simulink model "SingularityIdentification"  (R2022a)
settings: Solver=ode4  StartTime=0.0  StopTime=Inf  FixedStep=1/500  RelTol=1e-3
InitFcn:
  | L1 = 0.1400;
  | L2 = 0.3500;
  | L3 = 0.0500;
  | L4 = 0.2500;
  | L5 = 0.1500;
  | l1 = L1;
  | l2 = sqrt(L2^2 + L3^2);
  | l3 = L4 + L5;
  | beta = atan(L3/L2);
  | 
  | home = [0.45; 0; 0.49];
  | default = home;
  | default_w = [0.25; 0.25; 0.1];
  | default_a = [0; 0.375; 0.1];
  | A = [ 0.25; 0.25; 0.01];
  | B = [ 0.25; 0.50; 0.01];
  | C = [-0.25; 0.50; 0.01];
  | D = [-0.25; 0.25; 0.01];
  | 
  | welding_waypoints = [default_w, A, B, C, D, A]' ;
  | assembly_waypoints = [default_a, A, default_a, B, default_a, C, default_a, D]' ;
  | 
  | waypoints = welding_waypoints;
undefined symbols (not defined in the file): HIL, Host
libraries: quarc_library x8
settings Model: ExtModeTrigDuration=10000  Creator=fvranes  LastModifiedBy=lgonzalez
settings SolverCC: AlgebraicLoopSolver=TrustRegion
settings DataIOCC: ReturnWorkspaceOutputs=off
settings DebuggingCC: UnderspecifiedInitializationDetection=Classic  MergeDetectMultiDrivingBlocksExec=none  UnconnectedInputMsg=warning  UnconnectedOutputMsg=warning  UnconnectedLineMsg=warning
settings ModelReferenceCC: PropagateSignalLabelsOutOfModel=off
settings SFSimCC: CustomCodeUndefinedFunction=UseInterfaceOnly

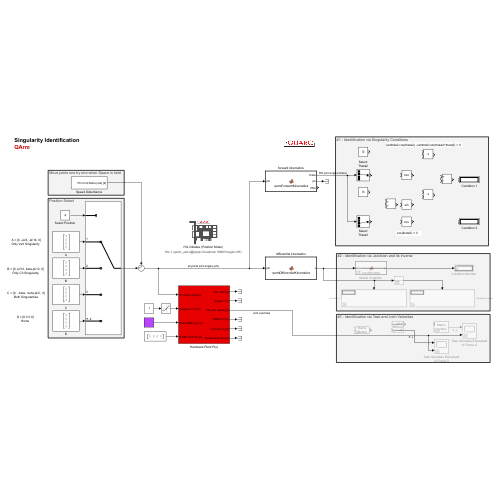
[thumbnail: Simulink's stored preview of the top-level diagram]
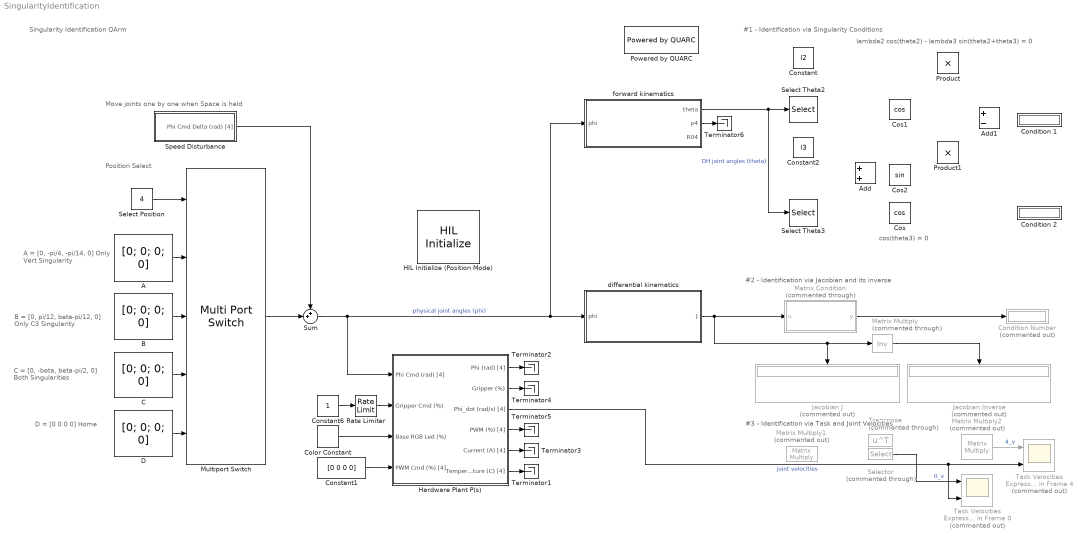
== system SingularityIdentification ==
  note: Move joints one by one when Space is held
  note: Position Select
  note: lambda2 cos(theta2) - lambda3 sin(theta2+theta3) = 0
  note: #1 - Identification via Singularity Conditions
  note: #3 - Identification via Task and Joint Velocities
  note: #2 - Identification via Jacobian and its inverse
  note: A = [0, -pi/4, -pi/14, 0]
      | Only Vert Singularity
  note: B = [0, pi/12, beta-pi/12, 0]
      | Only C3 Singularity
  note: C = [0, -beta, beta-pi/2, 0]
      | Both Singularities
  note: D = [0 0 0 0]
      | Home
  note: cos(theta3) = 0
  note: Singularity Identification
      | QArm
  A : Constant  Value=[0; 0; 0; 0]  VectorParams1D=off
  Add : Sum
  Add1 : Sum  Inputs=+-
  B : Constant  Value=[0; 0; 0; 0]  VectorParams1D=off
  C : Constant  Value=[0; 0; 0; 0]  VectorParams1D=off
  Color Constant : quarc_library/Sources/Signals/Color Constant  color=[0.71765 0.27451 1]
      settings: SourceProductName=QUARC Targets
  Condition 1 : Display
  Condition 2 : Display
  Condition Number : Display  Commented=on
  Constant : Constant  Value=l2
  Constant1 : Constant  Value=[0 0 0 0]
  Constant2 : Constant  Value=l3
  Constant6 : Constant
  Cos : Trigonometry  Operator=cos
  Cos1 : Trigonometry  Operator=cos
  Cos2 : Trigonometry
  D : Constant  Value=[0; 0; 0; 0]  VectorParams1D=off
  HIL Initialize (Position Mode) : quarc_library/Data Acquisition/Generic/Configuration/HIL Initialize  object_name=HIL-1  board_type=qarm_usb  board_number=0@tcpip://localhost:18900?nagle='off'  board_options=j0_mode=0;j1_mode=0;j2_mode=0;j3_mode=0;gripper_mode=0;  exclusive=off  active=on  hardware_clocks=[0]  clock_modes=[]  initial_clock_frequencies=[]  set_clock_params_at_start=off  set_clock_params_at_switch_in=off  set_clock_frequencies_at_start=off  set_clock_frequencies_at_switch_in=off  analog_input_channels=[5:9]  analog_input_configurations=[]  analog_input_maximums=[]  analog_input_minimums=[]  set_analog_input_params_at_start=off  set_analog_input_params_at_switch_in=off  analog_output_channels=[]  analog_output_maximums=inf  analog_output_minimums=-inf  initial_analog_outputs=[0]  final_analog_outputs=[0]  watchdog_analog_outputs=[]  set_analog_output_params_at_start=off  set_analog_output_params_at_switch_in=off  set_analog_outputs_at_start=off  set_analog_outputs_at_switch_in=off  set_analog_outputs_at_terminate=off  set_analog_outputs_at_switch_out=off  set_analog_outputs_on_watchdog=off  digital_input_channels=[]  digital_output_channels=[]  digital_output_configuration=[]  initial_digital_outputs=[0]  final_digital_outputs=[0]  watchdog_digital_outputs=[0]  set_digital_output_params_at_start=off  set_digital_output_params_at_switch_in=off  set_digital_outputs_at_start=off  set_digital_outputs_at_switch_in=off  set_digital_outputs_at_terminate=off  set_digital_outputs_at_switch_out=off  set_digital_outputs_on_watchdog=off  encoder_channels=[]  quadrature=[]  encoder_filter_frequency=[]  initial_encoder_counts=[]  set_encoder_params_at_start=off  set_encoder_params_at_switch_in=off  set_encoder_counts_at_start=off  set_encoder_counts_at_switch_in=off  pwm_channels=[]  pwm_modes=[]  pwm_frequency=[]  pwm_configuration=[]  pwm_alignment=[]  pwm_polarity=[]  pwm_leading_deadband=[]  pwm_trailing_deadband=[]  initial_pwm_outputs=[]  final_pwm_outputs=[]  watchdog_pwm_outputs=[]  set_pwm_params_at_start=off  set_pwm_params_at_switch_in=off  set_pwm_outputs_at_start=off  set_pwm_outputs_at_switch_in=off  set_pwm_outputs_at_terminate=off  set_pwm_outputs_at_switch_out=off  set_pwm_outputs_on_watchdog=off  other_output_channels=[1000:1004 11000:11003 11005:11007]  initial_other_outputs=[zeros(1,9), ones(1,3)]  final_other_outputs=[zeros(1,9), ones(1,3)]  watchdog_other_outputs=zeros(1,12)  set_other_outputs_at_start=off  set_other_outputs_at_switch_in=off  set_other_outputs_at_terminate=on  set_other_outputs_at_switch_out=off  set_other_outputs_on_watchdog=off
  Hardware Plant P(s) : Subsystem
  Jacobian Inverse : Display  Commented=on
  Jacobian J : Display  Commented=on
  Matrix Condition : MATLAB Function  Commented=through  TreatAsAtomicUnit=on
  Matrix Multiply : Product  Commented=through  Inputs=/  Multiplication=Matrix(*)
  Matrix Multiply1 : Product  Commented=on  Multiplication=Matrix(*)
  Matrix Multiply2 : Product  Commented=on  Multiplication=Matrix(*)
  Multiport Switch : MultiPortSwitch  Inputs=4  SaturateOnIntegerOverflow=off  InputSameDT=off
  Powered by QUARC : quarc_library/Logos/Powered by QUARC
  Product : Product
  Product1 : Product
  Rate Limiter : RateLimiter  SampleTimeMode=inherited
  Select Theta2 : Selector  InputPortWidth=4  IndexOptions=Index vector (dialog)  Indices=2  OutputSizes=1
  Select Theta3 : Selector  InputPortWidth=4  IndexOptions=Index vector (dialog)  Indices=3  OutputSizes=1
  Select Position : Constant  Value=4
  Selector : Selector  Commented=through  InputPortWidth=4  IndexOptions=Index vector (dialog)  Indices=[1:3]  OutputSizes=1
  Speed Disturbance : Subsystem
  Sum : Sum  Inputs=++|
  Task Velocities Expressed in Frame 0 : Scope  Commented=on  NumInputPorts=2
  Task Velocities Expressed in Frame 4 : Scope  Commented=on  NumInputPorts=2
  Terminator{1..6} (6 alike) : Terminator
  Transpose : Math  Commented=through  Operator=transpose  SignedPower=on
  differential kinematics : MATLAB Function  TreatAsAtomicUnit=on
  forward kinematics : MATLAB Function  TreatAsAtomicUnit=on
  wires:
  Hardware Plant P(s)/4(PWM (%) [4]) -> Terminator5/1
  Hardware Plant P(s)/3(Phi_dot (rad/s) [4]) -> Task Velocities Expressed in Frame 0/2, Task Velocities Expressed in Frame 4/2  "joint velocities"
  Hardware Plant P(s)/6(Temperature (C) [4]) -> Terminator1/1
  Sum/1 -> Hardware Plant P(s)/1(Phi Cmd (rad) [4]), forward kinematics/1(phi), differential kinematics/1(phi)  "physical joint angles (phi)"
  Rate Limiter/1 -> Hardware Plant P(s)/2(Gripper Cmd (%))
  Hardware Plant P(s)/5(Current (A) [4]) -> Terminator3/1
  Color Constant/1 -> Hardware Plant P(s)/3(Base RGB Led (%))
  Constant1/1 -> Hardware Plant P(s)/4(PWM Cmd (%) [4])
  Constant6/1 -> Rate Limiter/1
  Hardware Plant P(s)/2(Gripper (%)) -> Terminator4/1
  differential kinematics/1(J) -> Matrix Condition/1(u), Matrix Multiply/1, Jacobian J/1
  Speed Disturbance/1(Phi Cmd Delta (rad) [4]) -> Sum/1
  Multiport Switch/1 -> Sum/2
  C/1 -> Multiport Switch/4
  B/1 -> Multiport Switch/3
  A/1 -> Multiport Switch/2
  Select Position/1 -> Multiport Switch/1
  D/1 -> Multiport Switch/5
  forward kinematics/1(theta) -> Select Theta3/1, Select Theta2/1  "DH joint angles (theta)"
  Hardware Plant P(s)/1(Phi (rad) [4]) -> Terminator2/1
  forward kinematics/2(p4) -> Terminator6/1
  Matrix Multiply2/1 -> Task Velocities Expressed in Frame 4/1  "4_v"
  Selector/1 -> Task Velocities Expressed in Frame 0/1  "0_v"
  Matrix Multiply/1 -> Jacobian Inverse/1
  Matrix Condition/1(y) -> Condition Number/1

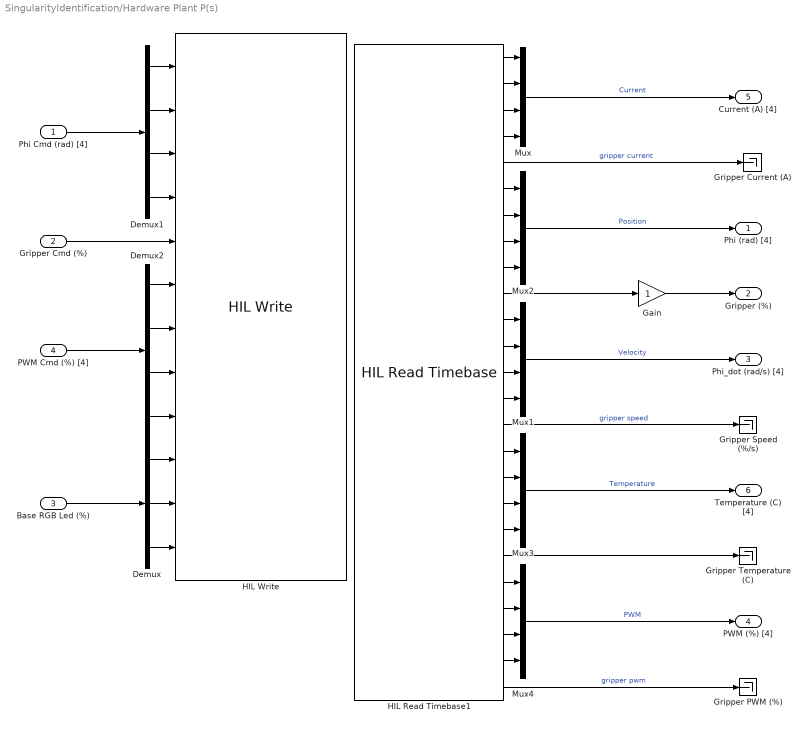
== system SingularityIdentification/Hardware Plant P(s) ==
  Phi Cmd (rad) [4] : Inport
  Gripper Cmd (%) : Inport  Port=2
  Base RGB Led (%) : Inport  Port=3
  PWM Cmd (%) [4] : Inport  Port=4
  Demux : Demux  Outputs=3
  Demux1 : Demux
  Demux2 : Demux
  Gain : Gain
  Gripper Current (A) : Terminator
  Gripper PWM (%) : Terminator
  Gripper Speed (%/s) : Terminator
  Gripper Temperature (C) : Terminator
  HIL Read Timebase1 : quarc_library/Data Acquisition/Generic/Timebases/HIL Read Timebase  object_name=HIL-1  clock=0  analog_channels=[5:9]  encoder_channels=[]  digital_channels=[]  other_channels=[1000:1004 3000:3004 10000:10004 11000:11004]  active=on  vector_output=off  data_type_mode=Inherit via back propagation  encoder_data_type=double  digital_data_type=boolean  overflow_mode=Synchronize (for simulated cards only)  samples_in_buffer=1
  HIL Write : quarc_library/Data Acquisition/Generic/Immediate I//O/HIL Write  object_name=HIL-1  analog_channels=[]  pwm_channels=[]  digital_channels=[]  other_channels=[1000:1004 11000:11003 11005:11007]  sample_time=-1  active=on  vector_input=off
  Mux{,1..4} (5 alike) : Mux
  Phi (rad) [4] : Outport  VectorParamsAs1DForOutWhenUnconnected=off
  Gripper (%) : Outport  Port=2  VectorParamsAs1DForOutWhenUnconnected=off
  Phi_dot (rad/s) [4] : Outport  Port=3  VectorParamsAs1DForOutWhenUnconnected=off
  PWM (%) [4] : Outport  Port=4  VectorParamsAs1DForOutWhenUnconnected=off
  Current (A) [4] : Outport  Port=5  VectorParamsAs1DForOutWhenUnconnected=off
  Temperature (C) [4] : Outport  Port=6  VectorParamsAs1DForOutWhenUnconnected=off
  wires:
  HIL Read Timebase1/14 -> Mux1/4
  HIL Read Timebase1/9 -> Mux2/4
  HIL Read Timebase1/6 -> Mux2/1
  HIL Read Timebase1/18 -> Mux3/3
  HIL Read Timebase1/8 -> Mux2/3
  HIL Read Timebase1/12 -> Mux1/2
  HIL Read Timebase1/4 -> Mux/4
  HIL Read Timebase1/7 -> Mux2/2
  HIL Read Timebase1/5 -> Gripper Current (A)/1  "gripper current"
  HIL Read Timebase1/15 -> Gripper Speed (%/s)/1  "gripper speed"
  Demux/3 -> HIL Write/12
  HIL Read Timebase1/3 -> Mux/3
  HIL Read Timebase1/17 -> Mux3/2
  HIL Read Timebase1/16 -> Mux3/1
  HIL Read Timebase1/11 -> Mux1/1
  Demux/1 -> HIL Write/10
  HIL Read Timebase1/19 -> Mux3/4
  Demux/2 -> HIL Write/11
  HIL Read Timebase1/13 -> Mux1/3
  HIL Read Timebase1/2 -> Mux/2
  HIL Read Timebase1/1 -> Mux/1
  HIL Read Timebase1/20 -> Gripper Temperature (C)/1
  Mux/1 -> Current (A) [4]/1  "Current"
  Mux1/1 -> Phi_dot (rad/s) [4]/1  "Velocity"
  Mux3/1 -> Temperature (C) [4]/1  "Temperature"
  Base RGB Led (%)/1 -> Demux/1
  Demux1/1 -> HIL Write/1
  Demux1/2 -> HIL Write/2
  Demux1/3 -> HIL Write/3
  Demux1/4 -> HIL Write/4
  Phi Cmd (rad) [4]/1 -> Demux1/1
  PWM Cmd (%) [4]/1 -> Demux2/1
  Demux2/1 -> HIL Write/6
  Demux2/2 -> HIL Write/7
  Demux2/3 -> HIL Write/8
  Demux2/4 -> HIL Write/9
  Mux2/1 -> Phi (rad) [4]/1  "Position"
  HIL Read Timebase1/21 -> Mux4/1
  HIL Read Timebase1/22 -> Mux4/2
  HIL Read Timebase1/23 -> Mux4/3
  HIL Read Timebase1/24 -> Mux4/4
  HIL Read Timebase1/25 -> Gripper PWM (%)/1  "gripper pwm"
  Mux4/1 -> PWM (%) [4]/1  "PWM"
  HIL Read Timebase1/10 -> Gain/1
  Gain/1 -> Gripper (%)/1
  Gripper Cmd (%)/1 -> HIL Write/5

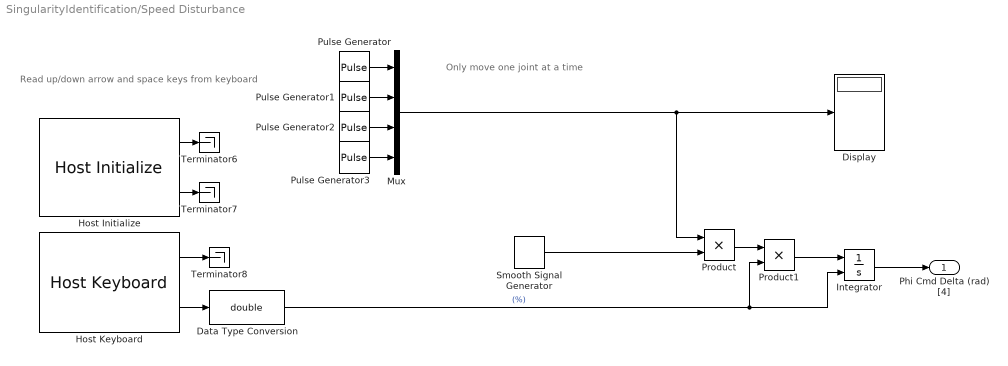
== system SingularityIdentification/Speed Disturbance ==
  note: Only move one joint at a time
  note: Read up/down arrow and space keys from keyboard
  Data Type Conversion : DataTypeConversion  OutDataTypeStr=double  SaturateOnIntegerOverflow=off  RndMeth=Floor
  Display : Display
  Host Initialize : quarc_library/Devices/Peripherals/Host/Host Initialize  object_name=Host-1  uri_source=Use external mode communications  uri=tcpip://localhost:18001  send_buffer_size=1000  receive_buffer_size=1000  thread_priority=0  run_client=on  use_window=off  window_position=[]  sample_time=qc_get_step_size  active=on
      settings: SourceProductName=QUARC Targets
  Host Keyboard : quarc_library/Devices/Peripherals/Host/Host Keyboard  object_name=Host-1  virtual_key=[32]  sample_time=qc_get_step_size  enabled=on  debug_mode=off
      settings: SourceProductName=QUARC Targets
  Integrator : Integrator  ExternalReset=either  InitialCondition=[0 0 0 0]
  Mux : Mux
  Product : Product
  Product1 : Product
  Pulse Generator : DiscretePulseGenerator  PulseType=Time based  Period=8  PulseWidth=25
  Pulse Generator1 : DiscretePulseGenerator  PulseType=Time based  Period=8  PulseWidth=25  PhaseDelay=2
  Pulse Generator2 : DiscretePulseGenerator  PulseType=Time based  Period=8  PulseWidth=25  PhaseDelay=4
  Pulse Generator3 : DiscretePulseGenerator  PulseType=Time based  Period=8  PulseWidth=25  PhaseDelay=6
  Smooth Signal Generator : quarc_library/Sources/Signals/Smooth Signal Generator  signal_type=Sine  source=Internal (dialog parameters)  amplitude=3*pi/180  frequency=1  initial_phase=0  sample_time=qc_get_step_size  output_cos=off
      settings: SourceProductName=QUARC Targets
  Terminator6 : Terminator
  Terminator7 : Terminator
  Terminator8 : Terminator
  Phi Cmd Delta (rad) [4] : Outport  VectorParamsAs1DForOutWhenUnconnected=off
  wires:
  Host Keyboard/1 -> Terminator8/1
  Host Initialize/2 -> Terminator7/1
  Host Initialize/1 -> Terminator6/1
  Host Keyboard/2 -> Data Type Conversion/1
  Product1/1 -> Integrator/1
  Mux/1 -> Product/1, Display/1
  Smooth Signal Generator/1 -> Product/2
  Data Type Conversion/1 -> Integrator/2, Product1/2  "(%)"
  Product/1 -> Product1/1
  Integrator/1 -> Phi Cmd Delta (rad) [4]/1
  Pulse Generator1/1 -> Mux/2
  Pulse Generator/1 -> Mux/1
  Pulse Generator2/1 -> Mux/3
  Pulse Generator3/1 -> Mux/4

== matlab function SingularityIdentification/differential kinematics ==
  data: phi input; J output
function J   = qarmDifferentialKinematics(phi)

%% QUANSER_ARM_FDK
% v 1.0 - 13th August 2020

% REFERENCE: 
% Chapter 5. Velocity Kinematics
% Robot Dynamics and Control 
% Spong, Vidyasagar
% 1989

% INPUTS:
% phi     : Alternate joint angles vector 4 x 1

% OUTPUTS:
% p4      : End-effector frame {4} position vector expressed in base frame {0}
% R04     : rotation matrix from end-effector frame {4} to base frame {0}

%% Manipulator parameters:
L1 = 0.1400;
L2 = 0.3500;
L3 = 0.0500;
L4 = 0.2500;
L5 = 0.1500;

%% Alternate parameters
l1 = L1;
l2 = sqrt(L2^2 + L3^2);
l3 = L4 + L5;
beta = atan(L3/L2);

%% From phi space to theta space 
theta = phi;
theta(1) = phi(1);
theta(2) = phi(2) + beta - pi/2;
theta(3) = phi(3) - beta;
theta(4) = phi(4);

%% Jacobian term definition:

J = eye(4);
J(1,1) = ; 
J(1,2) = ; 
J(1,3) = ; 
J(1,4) = ;
J(2,1) = ; 
J(2,2) = ;
J(2,3) = ;
J(2,4) = ;
J(3,1) = ;
J(3,2) = ;
J(3,3) = ;
J(3,4) = ;
J(4,1) = ;
J(4,2) = ;
J(4,3) = ;
J(4,4) = ;

end

== matlab function SingularityIdentification/forward kinematics ==
  data: theta output; phi input; p4 output; R04 output
function [theta, p4, R04] = qarmForwardKinematics(phi)

%% QUANSER_ARM_FPK
% v 4.0 - 4th June 2020

% REFERENCE: 
% Chapter 3. Forward Kinematics
% Robot Dynamics and Control 
% Spong, Vidyasagar
% 1989

% INPUTS:
% phi     : Alternate joint angles vector 4 x 1

% OUTPUTS:
% p4      : End-effector frame {4} position vector expressed in base frame {0}
% R04     : rotation matrix from end-effector frame {4} to base frame {0}

%% Manipulator parameters:
L1 = 0.1400;
L2 = 0.3500;
L3 = 0.0500;
L4 = 0.2500;
L5 = 0.1500;

%% Alternate parameters
l1 = ;
l2 = ;
l3 = ;
beta = ;

%% From phi space to theta space 
theta = phi;
theta(1) = phi(1);
theta(2) = phi(2);
theta(3) = phi(3);
theta(4) = phi(4);

%% Transformation matrices for all frames:

% T{i-1}{i} = quanser_arm_DH(  a, alpha,  d,     theta );
        T01 = quanser_arm_DH(  0,     0,  0,         0 );
        T12 = quanser_arm_DH(  0,     0,  0,         0 );
        T23 = quanser_arm_DH(  0,     0,  0,         0 );
        T34 = quanser_arm_DH(  0,     0,  0,         0 );

        T02 = ;
        T03 = ;
        T04 = ;

%% Position of end-effector Transformation

% Extract the Position vector 
p4 = ;

% Extract the Rotation matrix
R04 = ;

end

function T = quanser_arm_DH(a,alpha,d,theta)

%% QUANSER_ARM_DH
% v 1.0 - 26th March 2019

% REFERENCE: 
% Chapter 3. Forward and Inverse Kinematics
% Robot Modeling and Control 
% Spong, Hutchinson, Vidyasagar
% 2006

% INPUTS:
% a       :   translation  : along : x_{i}   : from : z_{i-1} : to : z_{i}
% alpha   :      rotation  : about : x_{i}   : from : z_{i-1} : to : z_{i}
% d       :   translation  : along : z_{i-1} : from : x_{i-1} : to : x_{i}
% theta   :      rotation  : about : z_{i-1} : from : x_{i-1} : to : x_{i}
% NOTE: Standard DH Parameters

% OUTPUTS:
% T       : transformation                   : from :     {i} : to : {i-1}

%%
% Rotation Transformation about z axis by theta
T_R_z = ;
     
% Translation Transformation along z axis by d
T_T_z = ;

% Translation Transformation along x axis by a
T_T_x = ;

% Rotation Transformation about x axis by alpha
T_R_x = ;

% For a transformation FROM frame {i} TO frame {i-1}: A
% rotate about x, 
% then translate along x, 
% then translate along z, 
% lastly, rotate about z
T = ;

end

== matlab function SingularityIdentification/Matrix Condition ==
  data: u input; y output
% Determine the condition number of a matrix

function y = condNumber(u)
y = cond(u);
